simulink model "customPVA"  (R2017b)
settings: Solver=ode23t  StartTime=0.0  StopTime=6  FixedStep=0.0001  MinStep=1e-14  RelTol=1e-10
StopFcn:
  | run('plot_IV_curve')
undefined symbols (not defined in the file or in its folder): E, physconst, T
libraries: powerlib x5, simulink x2
settings Model: Creator=Adrian  LastModifiedBy=Adrian
settings SolverCC: MaxConsecutiveMinStep=4  SolverJacobianMethodControl=FullPerturbation

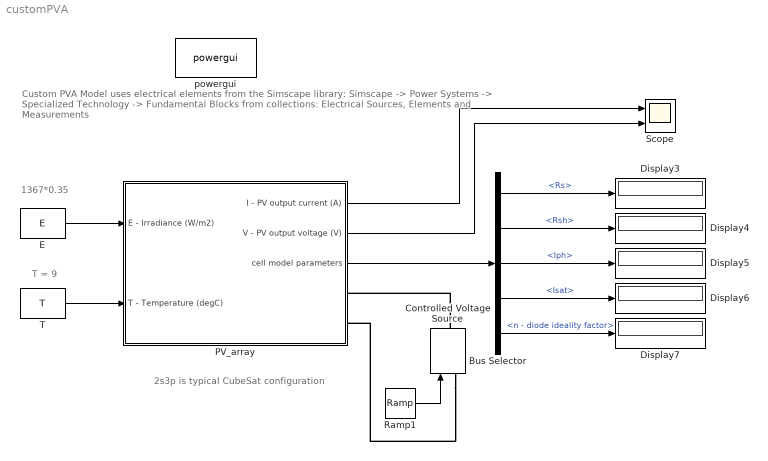
== system customPVA ==
  note: 2s3p is typical CubeSat configuration
  note: T = 9
  note: 1367*0.35
  note: Custom PVA
      | Model uses electrical elements from the Simscape library:
      | Simscape -> Power Systems -> Specialized Technology -> Fundamental Blocks
      | from collections: Electrical Sources, Elements and Measurements
  Bus Selector : BusSelector  OutputSignals=Rs,Rsh,Iph,Isat,n - diode ideality factor
  Controlled Voltage Source : powerlib/Electrical Sources/Controlled Voltage Source  Initialize=off  Source_Type=DC  Amplitude=0  Phase=0  Frequency=0  Measurements=None
  Display{3..7} (5 alike) : Display
  E : Constant  Value=E
  PV_array : Subsystem  mask(PV Array Model){s=2, p=3, n=2.5, T_ref=28, E_ref=1367, Voc_ref=2690, Isc_ref=519.6, Vmp_ref=2409, Imp_ref=502.9, kVoc=-6.2, kIsc=0.36, kVmp=-6.7, kImp=0.24}
      mask prompts: s "Serial cells (s)"; p "Parallel cells (p)"; n "Diode ideality factor / emission coefficient (n)"; T_ref "Temperature (degC), T_ref"; E_ref "Irradiation (W/m2), E_ref"; Voc_ref "Open circuit voltage (mV), Voc"; Isc_ref "Short circuit current (mA), Isc"; Vmp_ref "Voltage @ mpp (mV), Vmp"; Imp_ref "Current @ mpp (mA), Imp"; kVoc "Delta Voc / Delta T (mV/degC), kVoc"; kIsc "Delta Isc / Delta T (mA/degC), kIsc"; kVmp "Delta Vmp / Delta T (mV/degC), kVmp"; kImp "Delta Imp / Delta T (mA/degC), kImp"
      mask help:
      | This block models a PVA through the single diode solar cell model, scaled by the number of serial (s) and parallel (p) cells.
      | The diode ideality factor (n) of the model must be chosen. Reasonable values for n are 1.5 ... 2.5.
      | - Input: irradiance, cell temperature
      | - Output: electrical connections (current/voltage)
      mask init:
      | %% Input parameters for determination of 'Rs' initial guess
      | T_in = 0;      % [deg C] - Temperature (typical cell temperature)
      | 
      | %% Constants
      | k = 1.38064852e-23;          % [J/K] - Boltzmann constant
      | q = 1.6021766208e-19;        % [As]  - Elementary charge
      | 
      | %% Calculations
      | % Temperature dependent quantities
      | Vt = 1000*k*(T_in+273.15)/q;   % [mV] - thermal voltage
      | Isc = Isc_ref + (T_in - T_ref) * kIsc;
      | Voc = Voc_ref + (T_in - T_ref) * kVoc;
      | Imp = Imp_ref + (T_in - T_ref) * kImp;
      | Vmp = Vmp_ref + (T_in - T_ref) * kVmp;
      | % Determining Rs
      | n_diode = n;
      | syms Rs_sym
      | Term1 = simplify((n_diode*Vt*Vmp*(2*Imp-Isc))/((Vmp*Isc+Voc*(Imp-Isc))*(Vmp-Imp*Rs_sym)-n_diode*Vt*(Vmp*Isc-Voc*Imp)), 'Steps', 100);
      | Term2 = simplify(exp((Vmp+Imp*Rs_sym-Voc)/(n_diode*Vt)), 'Steps', 100);
      | Rs_sym = solve(Term1==Term2, Rs_sym);
      | Rs = double(Rs_sym);
      | 
      | % Set Rs as initial guess in solver block
      | set_param([gcb '/get_5_model_parameters/get_Rs/solve_Rs'], 'z0', num2str(Rs));
      mask Help:
      | - Input: irradiance, cell temperature
      | - Output: electrical connections (current/voltage)
      | 
      | - Single diode solar cell model
      | - Setup: current source, parallel diode, shunt and series resistor
      | - Block parameters are the solar cell data sheet values
      | - Model determines the 5 parameters of the single diode solar cell model (Iph, Isat, n, Rsh, Rs, where n must be chosen) using the block inputs and the block parameters, based on the approach of Villalva et al., 2009
      | - The 5 calculated model parameters are used to control an internal parametrized current source
      | - Model parameters are determined using Voc, Isc, V and I @ MPP and the corresponding temperature dependencies of the modeled solar cell as given in the data sheet
      | 
      | - n: Diode ideality factor (1.5...2.5 for reasonable results)
      | 
      | - CAUTION: when choosing a higher ideality factor (n) and/or when applying extreme temperatures, the modeled shunt resistance may result in a negative value. This is not critical, as the model does not claim to correspond to reality, only to depict it. However, this can be prevented by reducing (n).
      mask TypeOptions s: serial_cells/Value
      mask TypeOptions p: parallel_cells/Value
      mask TypeOptions n: get_5_model_parameters/n
      mask TypeOptions T_ref: get_5_model_parameters/T_ref
      mask TypeOptions E_ref: get_5_model_parameters/E_ref
      mask TypeOptions Voc_ref: get_5_model_parameters/Voc_ref
      mask TypeOptions Isc_ref: get_5_model_parameters/Isc_ref
      mask TypeOptions Vmp_ref: get_5_model_parameters/Vmp_ref
      mask TypeOptions Imp_ref: get_5_model_parameters/Imp_ref
      mask TypeOptions kVoc: get_5_model_parameters/kVoc
      mask TypeOptions kIsc: get_5_model_parameters/kIsc
      mask TypeOptions kVmp: get_5_model_parameters/kVmp
      mask TypeOptions kImp: get_5_model_parameters/kImp
      mask DialogControl Container5 Prompt: PV Array Configuration
      mask DialogControl Container9 Prompt: Model Parameterization
      mask DialogControl n Tooltip: Choose a valuue from 1.5 ... 2.5 for reasonable results
      mask DialogControl Container7 Prompt: Cell Parameters (as given in the data sheet)
      mask DialogControl ParameterGroupVar Prompt: Conditions of reference measurement
      mask DialogControl Container3 Prompt: Characteristics (reference measurement @ T_ref, E_ref)
      mask DialogControl Container4 Prompt: Temperature coefficients
  Ramp1 : simulink/Sources/Ramp  slope=1  start=0  X0=0
  Scope : Scope  NumInputPorts=2
  T : Constant  Value=T
  powergui : powerlib/powergui  Priority=1  SimulationMode=Discrete  SampleTime=1e-3  frequency=60  Iterations=50  frequencyindice=0  Pbase=100e6  ErrMax=1e-4  UnitsV=kV  UnitsW=MW  buscounter=0  FunctionMessages=off  echomessages=off  EnableUseOfTLC=off  CurrentSourceSwitches=off  DisableSnubberDevices=off  DisableRonSwitches=off  DisableVfSwitches=off  DisplayEquations=off  SolverType=Backward Euler  Interpol=off  ExternalGateDelay=off  methode=off  Ts=100  x0status=blocks  SPID=on  SwTol=0  HookPort=off  RestoreLinks=warning  ResistiveCurrentMeasurement=off  Frange=[0:2:500]  Ylog=off  Xlog=on  ShowGrid=off  save=off  variable=ZData  structure=0  ZoomFFT=off  StartTime=0.0  cycles=1  DisplayStyle=1  fundamental=60  FreqAxis=off  MaxFrequency=1000  frequencyindicesteady=1  RmsSteady=1  display=off
  wires:
  E/1 -> PV_array/1(E - Irradiance (W/m2))
  T/1 -> PV_array/2(T - Temperature (degC))
  PV_array/2(V - PV output voltage (V)) -> Scope/2
  PV_array/3(cell model parameters) -> Bus Selector/1
  Bus Selector/1 -> Display3/1  "<Rs>"
  Bus Selector/2 -> Display4/1  "<Rsh>"
  Bus Selector/3 -> Display5/1  "<Iph>"
  Bus Selector/4 -> Display6/1  "<Isat>"
  Bus Selector/5 -> Display7/1  "<n - diode ideality factor>"
  Ramp1/1 -> Controlled Voltage Source/1
  PV_array/1(I - PV output current (A)) -> Scope/1
  connections:
  Controlled Voltage Source/LConn1 -- PV_array/RConn2
  Controlled Voltage Source/RConn1 -- PV_array/RConn1

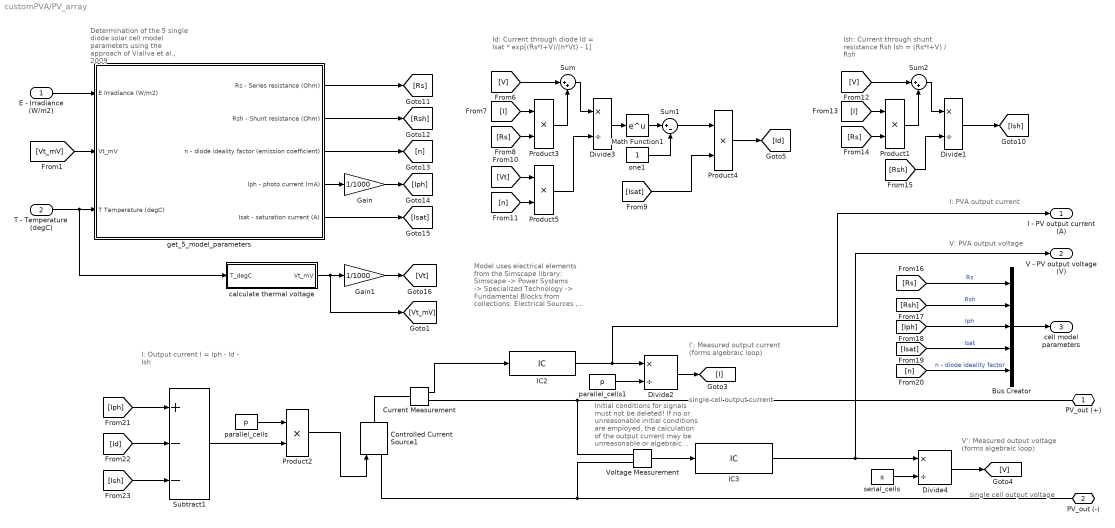
== system customPVA/PV_array ==
  note: single cell output current
  note: single cell output voltage
  note: Determination of the 5 single diode solar cell model parameters
      | using the approach of Viallva et al., 2009
  note: Id: Current through diode
      |
      | Id = Isat * exp[(Rs*I+V)/(n*Vt) - 1]
  note: Ish: Current through shunt resistance Rsh
      |
      | Ish = (Rs*I+V) / Rsh
  note: I': Measured output current
      | (forms algebraic loop)
  note: I: Output current
      |
      | I = Iph - Id - Ish
  note: V': Measured output voltage
      | (forms algebraic loop)
  note: Initial conditions for signals must not be deleted!
      | If no or unreasonable initial conditions are employed, the calculation of the
      | output current may be unreasonable or algebraic loops may not be solved.
  note: Model uses electrical elements from the Simscape library:
      | Simscape -> Power Systems -> Specialized Technology -> Fundamental Blocks
      | from collections: Electrical Sources , Elements and Measurements
  note: I: PVA output current
  note: V: PVA output voltage
  E - Irradiance (W/m2) : Inport
  T - Temperature (degC) : Inport  Port=2
  Bus Creator : BusCreator  Inputs=5
  Controlled Current Source1 : powerlib/Electrical Sources/Controlled Current Source  Initialize=on  Source_Type=DC  Amplitude=0  Phase=0  Frequency=0  Measurements=None
  Current Measurement : powerlib/Measurements/Current Measurement  PhasorSimulation=off  OutputType=Complex  PSBequivalent=0
  Divide{1..4} (4 alike) : Product  Inputs=*/
  Gain : Gain  Gain=1/1000
  Gain1 : Gain  Gain=1/1000
  IC2 : InitialCondition  Value=(Imp_ref*p)/1000
  IC3 : InitialCondition  Value=(Vmp_ref*s)/1000/2
  Math Function1 : Math  SaturateOnIntegerOverflow=on
  Product{1..5} (5 alike) : Product
  Subtract1 : Sum  Inputs=+--
  Sum : Sum  Inputs=|++
  Sum1 : Sum  Inputs=|+-
  Sum2 : Sum  Inputs=|++
  Voltage Measurement : powerlib/Measurements/Voltage Measurement  PhasorSimulation=off  OutputType=Complex  PSBequivalent=0
  calculate thermal voltage : Subsystem
  get_5_model_parameters : Subsystem  mask(Parameter identifier of "single diode" solar cell model){n=n, T_ref=T_ref, E_ref=E_ref, Voc_ref=Voc_ref, Isc_ref=Isc_ref, Vmp_ref=Vmp_ref, Imp_ref=Imp_ref, kVoc=kVoc, kIsc=kIsc, kVmp=kVmp, kImp=kImp}
      mask prompts: n "Diode ideality factor (emission coefficient)"; T_ref "Temperature (degC), T_ref ="; E_ref "Irradiation (W/m2), E_ref ="; Voc_ref "Open circuit voltage (mV), Voc"; Isc_ref "Short circuit current (mA), Isc"; Vmp_ref "Voltage @ mpp (mV), Vmp"; Imp_ref "Current @ mpp (mA), Imp"; kVoc "Delta Voc / Delta T (mV/degC), kVoc"; kIsc "Delta Isc / Delta T (mA/degC), kIsc"; kVmp "Delta Vmp / Delta T (mV/degC), kVmp"; kImp "Delta Imp / Delta T (mA/degC), kImp"
      mask help:
      | - solar cell model, type: single diode + innert losses
      | - using a current source, parallel diode, shunt and series resistor
      | - output: 5 parameters (Iph, Isat, n, Rsh, Rs)
      | - input: irradiance, temperature
      | - model parameters aret determined using Voc, Isc, V and I @ mpp and the corresponding temperature coefficients
      mask DialogControl Container5 Prompt: Tunable model parameters
      mask DialogControl n Tooltip: Choose a valuue from 1.5 ... 2.5 for reasonable results
      mask DialogControl ParameterGroupVar Prompt: Conditions of reference measurement
      mask DialogControl Container8 Prompt: Characteristics (reference measurement @ T_ref, E_ref)
      mask DialogControl Container9 Prompt: Temperature dependencies
  one1 : Constant
  parallel_cells : Constant  Value=p
  parallel_cells1 : Constant  Value=p
  serial_cells : Constant  Value=s
  PV_out (+) : PMIOPort  Port=1  Side=Right
  PV_out (-) : PMIOPort  Port=2  Side=Right
  I - PV output current (A) : Outport
  V - PV output voltage (V) : Outport  Port=2
  cell model parameters : Outport  Port=3
  wires:
  Gain/1 -> [Iph]
  [I] -> Product1/1
  Product1/1 -> Sum2/2
  [V] -> Sum2/1
  Divide3/1 -> Math Function1/1
  one1/1 -> Sum1/2
  Sum/1 -> Divide3/1
  [V] -> Sum/1
  Sum1/1 -> Product4/1
  [Rs] -> Product1/2
  Product3/1 -> Sum/2
  Math Function1/1 -> Sum1/1
  [Isat] -> Product4/2
  [Rsh] -> Divide1/2
  Product4/1 -> [Id]
  [Vt] -> Product5/1
  [n] -> Product5/2
  [I] -> Product3/1
  Product5/1 -> Divide3/2
  calculate thermal voltage/1(Vt_mV) -> [Vt_mV], Gain1/1
  get_5_model_parameters/4(Iph - photo current (mA)) -> Gain/1
  get_5_model_parameters/1(Rs - Series resistance (Ohm)) -> [Rs]
  get_5_model_parameters/5(Isat - saturation current (A)) -> [Isat]
  Sum2/1 -> Divide1/1
  Divide1/1 -> [Ish]
  get_5_model_parameters/2(Rsh - Shunt resistance (Ohm)) -> [Rsh]
  Gain1/1 -> [Vt]
  [Rs] -> Product3/2
  E - Irradiance (W/m2)/1 -> get_5_model_parameters/1(E Irradiance (W/m2))
  get_5_model_parameters/3(n - diode ideality factor (emission coefficient)) -> [n]
  IC3/1 -> Divide4/1, V - PV output voltage (V)/1
  [Rs] -> Bus Creator/1  "Rs"
  [Rsh] -> Bus Creator/2  "Rsh"
  [Iph] -> Bus Creator/3  "Iph"
  [Isat] -> Bus Creator/4  "Isat"
  Bus Creator/1 -> cell model parameters/1
  [n] -> Bus Creator/5  "n - diode ideality factor"
  Current Measurement/1 -> IC2/1
  [Ish] -> Subtract1/3
  [Id] -> Subtract1/2
  Voltage Measurement/1 -> IC3/1
  Subtract1/1 -> Product2/2
  parallel_cells/1 -> Product2/1
  Divide2/1 -> [I]
  Divide4/1 -> [V]
  Product2/1 -> Controlled Current Source1/1
  IC2/1 -> I - PV output current (A)/1, Divide2/1
  parallel_cells1/1 -> Divide2/2
  serial_cells/1 -> Divide4/2
  T - Temperature (degC)/1 -> get_5_model_parameters/3(T Temperature (degC)), calculate thermal voltage/1(T_degC)
  [Vt_mV] -> get_5_model_parameters/2(Vt_mV)
  [Iph] -> Subtract1/1
  connections:
  Controlled Current Source1/RConn1 -- Current Measurement/LConn1
  PV_out (-)/RConn1 -- Voltage Measurement/LConn2 -- Controlled Current Source1/LConn1
  Voltage Measurement/LConn1 -- PV_out (+)/RConn1 -- Current Measurement/RConn1

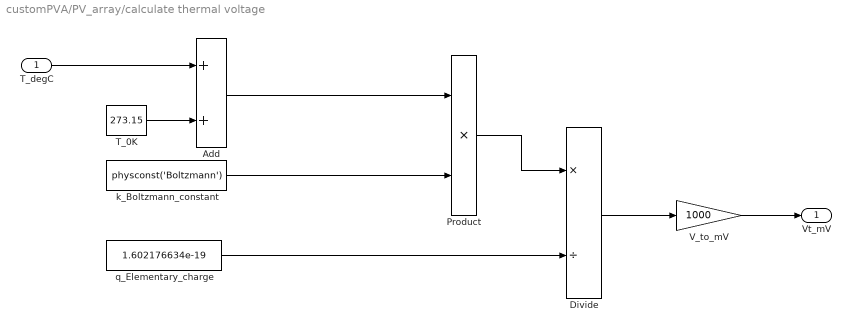
== system customPVA/PV_array/calculate thermal voltage ==
  T_degC : Inport
  Add : Sum
  Divide : Product  Inputs=*/
  Product : Product
  T_0K : Constant  Value=273.15
  V_to_mV : Gain  Gain=1000
  k_Boltzmann_constant : Constant  Value=physconst('Boltzmann')
  q_Elementary_charge : Constant  Value=1.602176634e-19
  Vt_mV : Outport
  wires:
  Product/1 -> Divide/1
  Divide/1 -> V_to_mV/1
  k_Boltzmann_constant/1 -> Product/2
  V_to_mV/1 -> Vt_mV/1
  q_Elementary_charge/1 -> Divide/2
  Add/1 -> Product/1
  T_degC/1 -> Add/1
  T_0K/1 -> Add/2

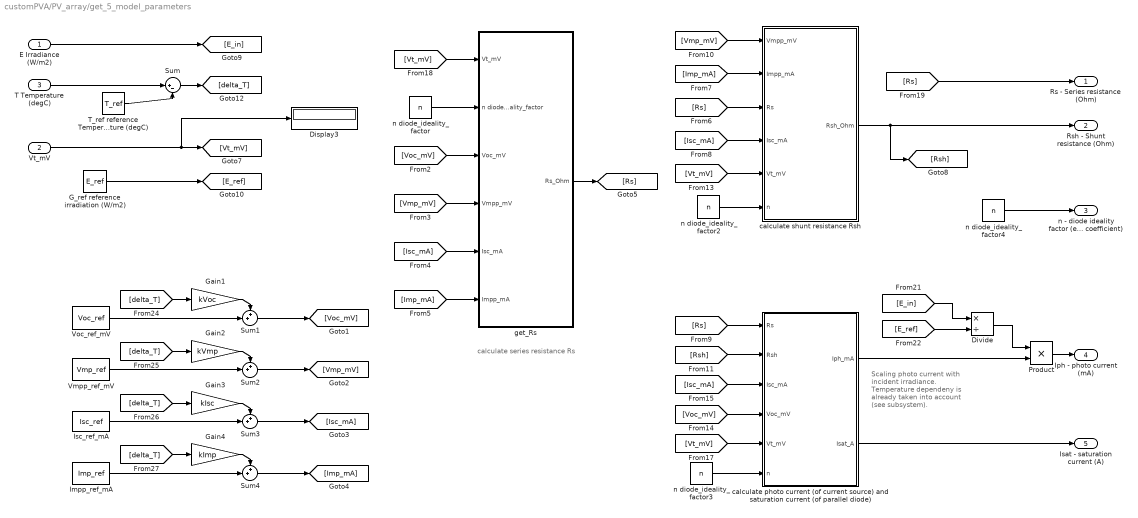
== system customPVA/PV_array/get_5_model_parameters ==
  note: calculate series resistance Rs
  note: Scaling photo current with incident irradiance.
      | Temperature dependeny is already taken into
      | account (see subsystem).
  E Irradiance (W/m2) : Inport
  Vt_mV : Inport  Port=2
  T Temperature (degC) : Inport  Port=3
  Display3 : Display
  Divide : Product  Inputs=*/
  G_ref reference irradiation (W/m2) : Constant  Value=E_ref
  Gain1 : Gain  Gain=kVoc
  Gain2 : Gain  Gain=kVmp
  Gain3 : Gain  Gain=kIsc
  Gain4 : Gain  Gain=kImp
  Impp_ref_mA : Constant  Value=Imp_ref
  Isc_ref_mA : Constant  Value=Isc_ref
  Product : Product
  Sum : Sum  Inputs=|+-
  Sum{1..4} (4 alike) : Sum  Inputs=++|
  T_ref reference Temperature (degC) : Constant  Value=T_ref
  Vmpp_ref_mV : Constant  Value=Vmp_ref
  Voc_ref_mV : Constant  Value=Voc_ref
  calculate photo current (of current source) and saturation current (of parallel diode) : Subsystem
  calculate shunt resistance Rsh : Subsystem
  get_Rs : Subsystem
  n diode_ideality_factor{,2..4} (4 alike) : Constant  Value=n
  Rs - Series resistance (Ohm) : Outport
  Rsh - Shunt resistance (Ohm) : Outport  Port=2
  n - diode ideality factor (emission coefficient) : Outport  Port=3
  Iph - photo current (mA) : Outport  Port=4
  Isat - saturation current (A) : Outport  Port=5
  wires:
  [Vt_mV] -> get_Rs/1(Vt_mV)
  [Imp_mA] -> get_Rs/6(Impp_mA)
  [Vmp_mV] -> get_Rs/4(Vmpp_mV)
  [Isc_mA] -> get_Rs/5(Isc_mA)
  [Voc_mV] -> get_Rs/3(Voc_mV)
  get_Rs/1(Rs_Ohm) -> [Rs]
  [Rs] -> calculate photo current (of current source) and saturation current (of parallel diode)/1(Rs)
  calculate photo current (of current source) and saturation current (of parallel diode)/2(Isat_A) -> Isat - saturation current (A)/1
  [Voc_mV] -> calculate photo current (of current source) and saturation current (of parallel diode)/4(Voc_mV)
  [Imp_mA] -> calculate shunt resistance Rsh/2(Impp_mA)
  [Vt_mV] -> calculate shunt resistance Rsh/5(Vt_mV)
  [Vt_mV] -> calculate photo current (of current source) and saturation current (of parallel diode)/5(Vt_mV)
  [Rs] -> calculate shunt resistance Rsh/3(Rs)
  [Isc_mA] -> calculate shunt resistance Rsh/4(Isc_mA)
  [Vmp_mV] -> calculate shunt resistance Rsh/1(Vmpp_mV)
  [Isc_mA] -> calculate photo current (of current source) and saturation current (of parallel diode)/3(Isc_mA)
  [Rsh] -> calculate photo current (of current source) and saturation current (of parallel diode)/2(Rsh)
  calculate shunt resistance Rsh/1(Rsh_Ohm) -> Rsh - Shunt resistance (Ohm)/1, [Rsh]
  T Temperature (degC)/1 -> Sum/1
  [Rs] -> Rs - Series resistance (Ohm)/1
  E Irradiance (W/m2)/1 -> [E_in]
  [E_in] -> Divide/1
  Product/1 -> Iph - photo current (mA)/1
  G_ref reference irradiation (W/m2)/1 -> [E_ref]
  [E_ref] -> Divide/2
  T_ref reference Temperature (degC)/1 -> Sum/2
  Sum/1 -> [delta_T]
  [delta_T] -> Gain1/1
  Voc_ref_mV/1 -> Sum1/2
  Gain1/1 -> Sum1/1
  Gain2/1 -> Sum2/1
  Vmpp_ref_mV/1 -> Sum2/2
  [delta_T] -> Gain2/1
  [delta_T] -> Gain4/1
  Impp_ref_mA/1 -> Sum4/2
  Gain4/1 -> Sum4/1
  Gain3/1 -> Sum3/1
  Isc_ref_mA/1 -> Sum3/2
  [delta_T] -> Gain3/1
  Sum1/1 -> [Voc_mV]
  Sum2/1 -> [Vmp_mV]
  Sum3/1 -> [Isc_mA]
  Sum4/1 -> [Imp_mA]
  Vt_mV/1 -> Display3/1, [Vt_mV]
  n diode_ideality_factor2/1 -> calculate shunt resistance Rsh/6(n)
  n diode_ideality_factor3/1 -> calculate photo current (of current source) and saturation current (of parallel diode)/6(n)
  n diode_ideality_factor4/1 -> n - diode ideality factor (emission coefficient)/1
  calculate photo current (of current source) and saturation current (of parallel diode)/1(Iph_mA) -> Product/2
  Divide/1 -> Product/1
  n diode_ideality_factor/1 -> get_Rs/2(n diode_ideality_factor)

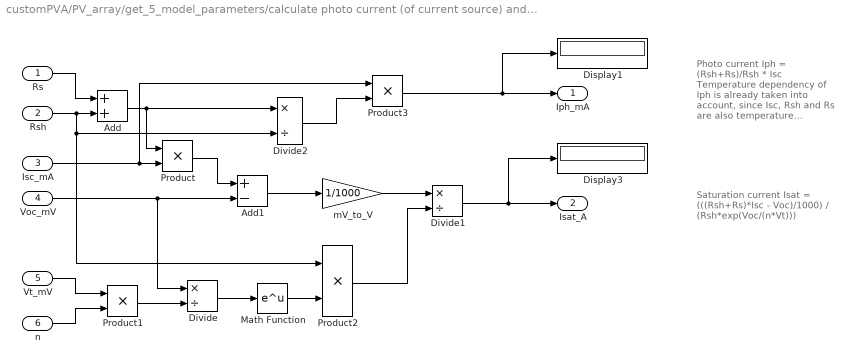
== system customPVA/PV_array/get_5_model_parameters/calculate photo current (of current source) and saturation current (of parallel diode) ==
  note: Saturation current
      | Isat = (((Rsh+Rs)*Isc - Voc)/1000) / (Rsh*exp(Voc/(n*Vt)))
  note: Photo current
      | Iph = (Rsh+Rs)/Rsh * Isc
      |
      | Temperature dependency of Iph is already taken into account,
      | since Isc, Rsh and Rs are also temperature dependent.
  Rs : Inport
  Rsh : Inport  Port=2
  Isc_mA : Inport  Port=3
  Voc_mV : Inport  Port=4
  Vt_mV : Inport  Port=5
  n : Inport  Port=6
  Add : Sum
  Add1 : Sum  Inputs=+-
  Display1 : Display
  Display3 : Display
  Divide : Product  Inputs=*/
  Divide1 : Product  Inputs=*/
  Divide2 : Product  Inputs=*/
  Math Function : Math  SaturateOnIntegerOverflow=on
  Product{,1..3} (4 alike) : Product
  mV_to_V : Gain  Gain=1/1000
  Iph_mA : Outport
  Isat_A : Outport  Port=2
  wires:
  Product2/1 -> Divide1/2
  Isc_mA/1 -> Product3/1, Product/2
  Divide/1 -> Math Function/1
  Voc_mV/1 -> Add1/2, Divide/1
  Product1/1 -> Divide/2
  Vt_mV/1 -> Product1/1
  Rs/1 -> Add/1
  Add1/1 -> mV_to_V/1
  n/1 -> Product1/2
  Divide1/1 -> Display3/1, Isat_A/1
  Product/1 -> Add1/1
  Rsh/1 -> Divide2/2, Product2/1, Add/2
  mV_to_V/1 -> Divide1/1
  Add/1 -> Product/1, Divide2/1
  Math Function/1 -> Product2/2
  Divide2/1 -> Product3/2
  Product3/1 -> Display1/1, Iph_mA/1

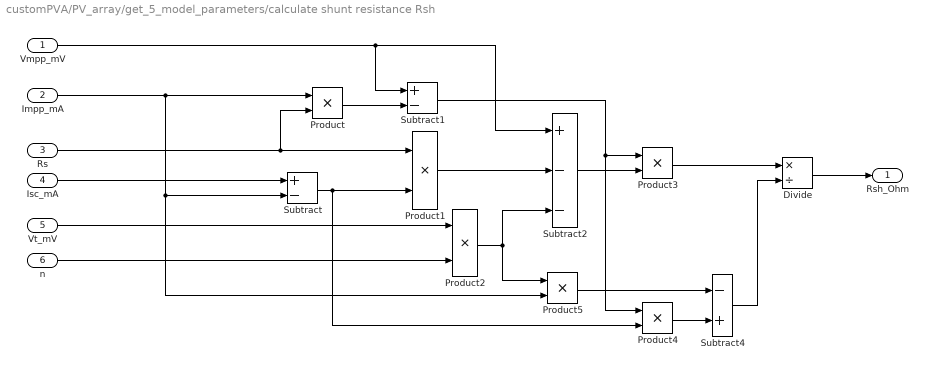
== system customPVA/PV_array/get_5_model_parameters/calculate shunt resistance Rsh ==
  Vmpp_mV : Inport
  Impp_mA : Inport  Port=2
  Rs : Inport  Port=3
  Isc_mA : Inport  Port=4
  Vt_mV : Inport  Port=5
  n : Inport  Port=6
  Divide : Product  Inputs=*/
  Product{,1..5} (6 alike) : Product
  Subtract : Sum  Inputs=+-
  Subtract1 : Sum  Inputs=+-
  Subtract2 : Sum  Inputs=+--
  Subtract4 : Sum  Inputs=-+
  Rsh_Ohm : Outport
  wires:
  Subtract4/1 -> Divide/2
  Product3/1 -> Divide/1
  Product5/1 -> Subtract4/1
  Rs/1 -> Product/2, Product1/1
  Isc_mA/1 -> Subtract/1
  Product1/1 -> Subtract2/2
  Vmpp_mV/1 -> Subtract1/1, Subtract2/1
  n/1 -> Product2/2
  Vt_mV/1 -> Product2/1
  Subtract1/1 -> Product4/1, Product3/1
  Divide/1 -> Rsh_Ohm/1
  Product2/1 -> Subtract2/3, Product5/1
  Subtract/1 -> Product1/2, Product4/2
  Product/1 -> Subtract1/2
  Subtract2/1 -> Product3/2
  Product4/1 -> Subtract4/2
  Impp_mA/1 -> Subtract/2, Product5/2, Product/1

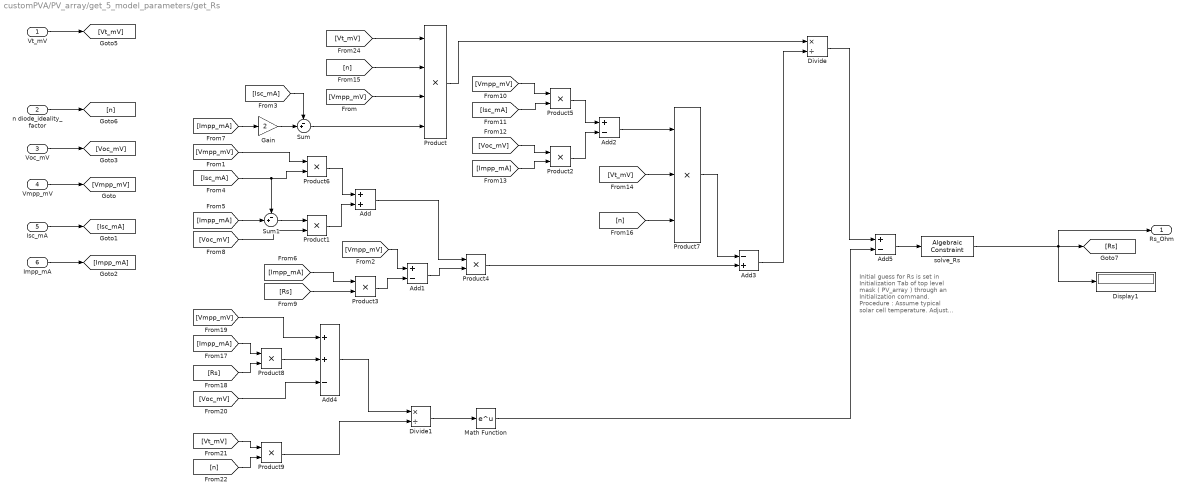
== system customPVA/PV_array/get_5_model_parameters/get_Rs ==
  note: Initial guess for Rs is set in Initialization Tab of top level mask
      | ( PV_array ) through an Initialization command.
      |
      | Procedure :
      | Assume typical solar cell temperature.
      | Adjust Voc, Isc, Vmp, Imp according to their temperature
      | coefficients and the solar cell temperature.
      | Determine Rs for chosen n value (diode emission factor set
      | through top level mask) using the approach of Villalva et al., 2009
      | with the Equations and systems solver from Matlab.
      | Set found Rs as initial guess parameter in the Simulink Algebraic
      | Constraints Block that solves for Rs during simulation.
  Vt_mV : Inport
  n diode_ideality_factor : Inport  Port=2
  Voc_mV : Inport  Port=3
  Vmpp_mV : Inport  Port=4
  Isc_mA : Inport  Port=5
  Impp_mA : Inport  Port=6
  Add : Sum
  Add1 : Sum  Inputs=+-
  Add2 : Sum  Inputs=+-
  Add3 : Sum  Inputs=-+
  Add4 : Sum  Inputs=++-
  Add5 : Sum  Inputs=+-
  Display1 : Display
  Divide : Product  Inputs=*/
  Divide1 : Product  Inputs=*/
  Gain : Gain  Gain=2
  Math Function : Math  SaturateOnIntegerOverflow=on
  Product : Product  Inputs=4
  Product{1..6,8..9} (8 alike) : Product
  Product7 : Product  Inputs=3
  Sum : Sum  Inputs=-+|
  Sum1 : Sum  Inputs=-+|
  solve_Rs : simulink/Math Operations/Algebraic Constraint  z0=0.087875
      settings: SourceProductName=Simulink  SourceProductBaseCode=SL
  Rs_Ohm : Outport
  wires:
  [Vmpp_mV] -> Add1/1
  Vmpp_mV/1 -> [Vmpp_mV]
  [Voc_mV] -> Add4/3
  Product7/1 -> Add3/1
  [Voc_mV] -> Product1/2
  [Vt_mV] -> Product/1
  [Voc_mV] -> Product2/1
  [Vmpp_mV] -> Add4/1
  Gain/1 -> Sum/2
  Product2/1 -> Add2/2
  [Vmpp_mV] -> Product/3
  Divide/1 -> Add5/1
  Product9/1 -> Divide1/2
  [n] -> Product/2
  [Vt_mV] -> Product7/2
  [Vmpp_mV] -> Product5/1
  [Impp_mA] -> Product8/1
  [Impp_mA] -> Sum1/2
  [Vmpp_mV] -> Product6/1
  Product5/1 -> Add2/1
  [Isc_mA] -> Sum/1
  [Impp_mA] -> Gain/1
  [Rs] -> Product3/2
  [n] -> Product7/3
  [Impp_mA] -> Product3/1
  Add/1 -> Product4/1
  Add2/1 -> Product7/1
  Divide1/1 -> Math Function/1
  n diode_ideality_factor/1 -> [n]
  Product1/1 -> Add/2
  Sum/1 -> Product/4
  [Vt_mV] -> Product9/1
  Add5/1 -> solve_Rs/1
  Add3/1 -> Divide/2
  [Isc_mA] -> Product5/2
  Product6/1 -> Add/1
  Vt_mV/1 -> [Vt_mV]
  Impp_mA/1 -> [Impp_mA]
  Isc_mA/1 -> [Isc_mA]
  Product3/1 -> Add1/2
  Sum1/1 -> Product1/1
  Voc_mV/1 -> [Voc_mV]
  Product8/1 -> Add4/2
  Add1/1 -> Product4/2
  Product/1 -> Divide/1
  [Rs] -> Product8/2
  [n] -> Product9/2
  [Impp_mA] -> Product2/2
  Add4/1 -> Divide1/1
  [Isc_mA] -> Sum1/1, Product6/2
  solve_Rs/1 -> Rs_Ohm/1, [Rs], Display1/1
  Math Function/1 -> Add5/2
  Product4/1 -> Add3/2
